simulink model "Lateral"  (R2024b)
settings: Solver=VariableStepAuto  StartTime=0.0  StopTime=10.0  RelTol=1e-3
settings Model: Creator=adam  LastModifiedBy=adam

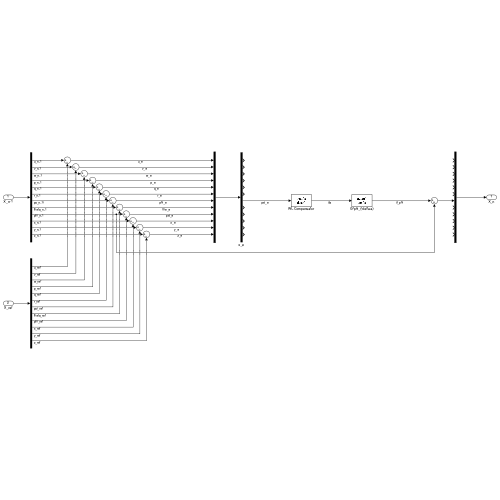
[thumbnail: Simulink's stored preview of the top-level diagram]
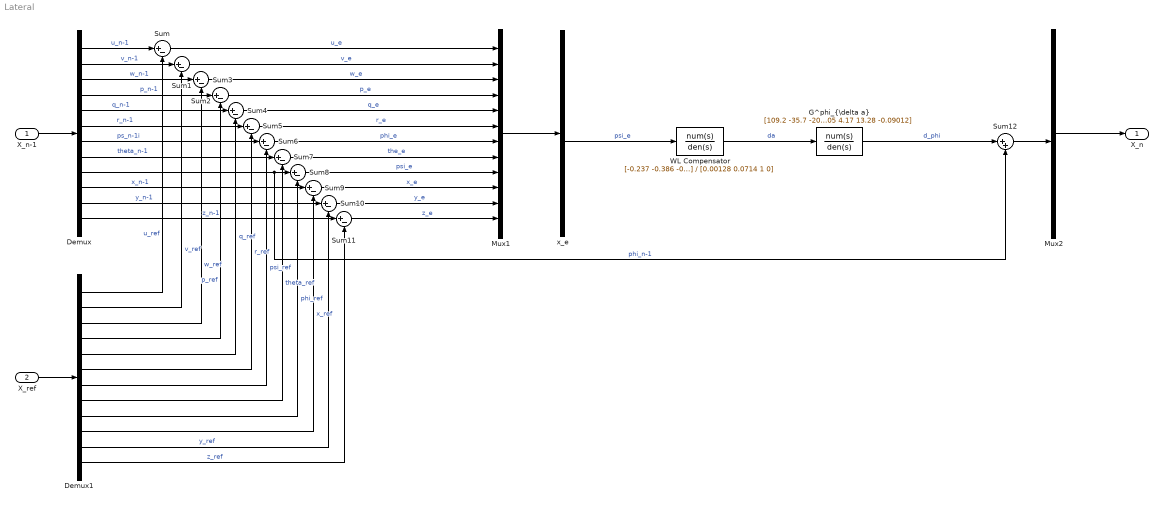
== system Lateral ==
  X_n-1 : Inport
  X_ref : Inport  Port=2
  Demux : Demux  Outputs=12
  Demux1 : Demux  Outputs=12
  "G^phi_{\\delta a}" : TransferFcn  Numerator=[109.2 -35.7 -206.3]  Denominator=[1 7.005 4.17 13.28 -0.09012]
  Mux1 : Mux  Inputs=12
  Mux2 : Mux  Inputs=12
  Sum{,1..11} (12 alike) : Sum  Inputs=|+-
  Sum12 : Sum  Inputs=|++
  WL Compensator : TransferFcn  Numerator=[-0.237 -0.386 -0.237]  Denominator=[0.00128 0.0714 1 0]
  x_e : Demux  Outputs=12
  X_n : Outport
  wires:
  X_n-1/1 -> Demux/1
  Demux/1 -> Sum/1  "u_n-1"
  Demux/12 -> Sum11/1  "z_n-1"
  Demux/11 -> Sum10/1  "y_n-1"
  Demux/10 -> Sum9/1  "x_n-1"
  Demux/8 -> Sum7/1  "theta_n-1"
  Demux/7 -> Sum6/1  "ps_n-1i"
  Demux/6 -> Sum5/1  "r_n-1"
  Demux/5 -> Sum4/1  "q_n-1"
  Demux/4 -> Sum3/1  "p_n-1"
  Demux/2 -> Sum1/1  "v_n-1"
  Demux/3 -> Sum2/1  "w_n-1"
  X_ref/1 -> Demux1/1
  Demux/9 -> Sum12/2, Sum8/1  "phi_n-1"
  Demux1/1 -> Sum/2  "u_ref"
  Sum/1 -> Mux1/1  "u_e"
  Demux1/2 -> Sum1/2  "v_ref"
  Sum1/1 -> Mux1/2  "v_e"
  Sum2/1 -> Mux1/3  "w_e"
  Demux1/3 -> Sum2/2  "w_ref"
  Demux1/4 -> Sum3/2  "p_ref"
  Sum3/1 -> Mux1/4  "p_e"
  Demux1/5 -> Sum4/2  "q_ref"
  Demux1/6 -> Sum5/2  "r_ref"
  Demux1/7 -> Sum6/2  "psi_ref"
  Demux1/8 -> Sum7/2  "theta_ref"
  Demux1/9 -> Sum8/2  "phi_ref"
  Demux1/10 -> Sum9/2  "x_ref"
  Demux1/11 -> Sum10/2  "y_ref"
  Demux1/12 -> Sum11/2  "z_ref"
  Mux1/1 -> x_e/1
  Sum11/1 -> Mux1/12  "z_e"
  Sum10/1 -> Mux1/11  "y_e"
  Sum9/1 -> Mux1/10  "x_e"
  Sum8/1 -> Mux1/9  "psi_e"
  Sum7/1 -> Mux1/8  "the_e"
  Sum6/1 -> Mux1/7  "phi_e"
  Sum5/1 -> Mux1/6  "r_e"
  Sum4/1 -> Mux1/5  "q_e"
  x_e/7 -> WL Compensator/1  "psi_e"
  WL Compensator/1 -> "G^phi_{\\delta a}"/1  "da"
  "G^phi_{\\delta a}"/1 -> Sum12/1  "d_phi"
  Mux2/1 -> X_n/1
  Sum12/1 -> Mux2/7
